simulink model "Unipolar_Bipolar_Sine_PWM_inverter"  (R2024b)
settings: Solver=VariableStepAuto  StartTime=0.0  StopTime=100e-3  RelTol=1e-3
libraries: spsMosfetLib x8, spsDCVoltageSourceLib x2, spsSeriesRLCBranchLib x2, spsTriangleGeneratorLib x2, spsVoltageMeasurementLib x2, sps_lib x1
settings Model: Creator=PRASHANTH  LastModifiedBy=PRASHANTH
settings DataIOCC: SaveOutput=off  SignalLogging=off  DSMLogging=off  ReturnWorkspaceOutputs=off  LoggingToFile=on

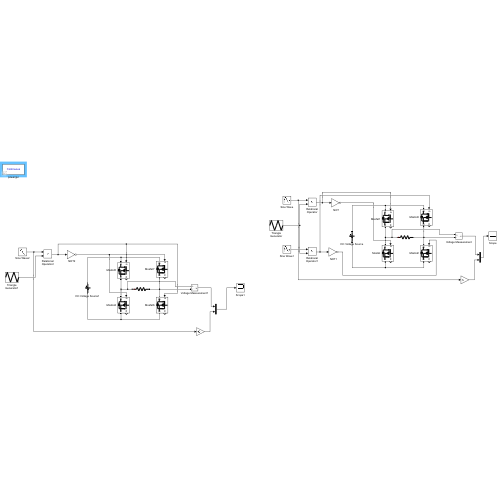
[thumbnail: Simulink's stored preview of the top-level diagram]
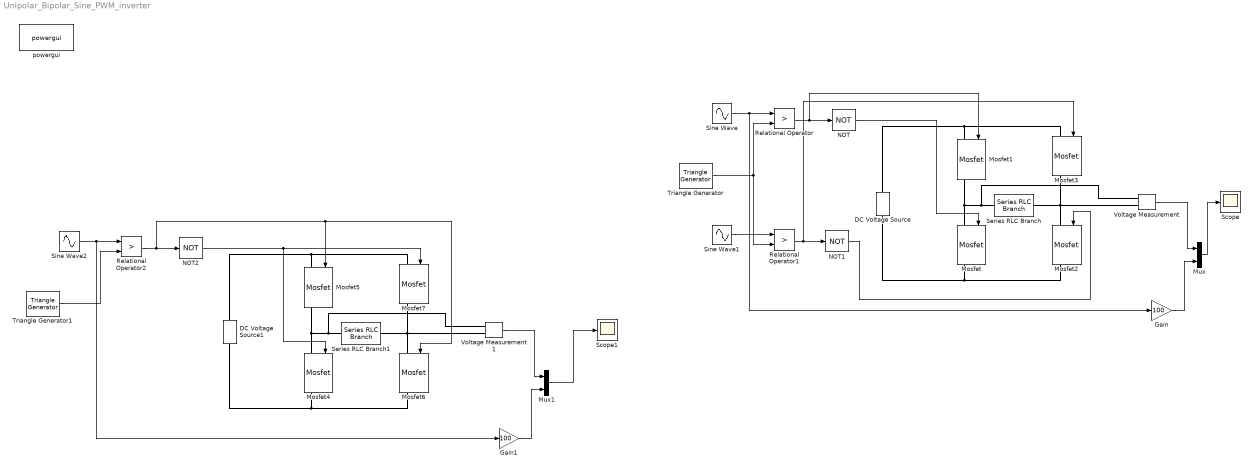
== system Unipolar_Bipolar_Sine_PWM_inverter ==
  DC Voltage Source : spsDCVoltageSourceLib/DC Voltage Source  Amplitude=100  Measurements=None
  DC Voltage Source1 : spsDCVoltageSourceLib/DC Voltage Source  Amplitude=100  Measurements=None
  Gain : Gain  Gain=100
  Gain1 : Gain  Gain=100
  Mosfet{,1..7} (8 alike) : spsMosfetLib/Mosfet  Ron=0.1  Lon=0  Rd=0.01  Vfd=0  IC=0  Rs=1e5  Cs=inf  Measurements=on
  Mux : Mux  Inputs=2
  Mux1 : Mux  Inputs=2
  NOT : Logic  Operator=NOT  IconShape=distinctive  AllPortsSameDT=off  OutDataTypeStr=boolean
  NOT1 : Logic  Operator=NOT  IconShape=distinctive  AllPortsSameDT=off  OutDataTypeStr=boolean
  NOT2 : Logic  Operator=NOT  IconShape=distinctive  AllPortsSameDT=off  OutDataTypeStr=boolean
  Relational Operator : RelationalOperator  Operator=>  OutDataTypeStr=boolean  RndMeth=Simplest  InputSameDT=off
  Relational Operator1 : RelationalOperator  Operator=>  OutDataTypeStr=boolean  RndMeth=Simplest  InputSameDT=off
  Relational Operator2 : RelationalOperator  Operator=>  OutDataTypeStr=boolean  RndMeth=Simplest  InputSameDT=off
  Scope : Scope
  Scope1 : Scope
  Series RLC Branch : spsSeriesRLCBranchLib/Series RLC Branch  LConnTagsString=__new0  RConnTagsString=__new0  BranchType=R  Resistance=10  Inductance=1e-3  SetiL0=off  InitialCurrent=0  Capacitance=1e-6  Setx0=off  InitialVoltage=0  Measurements=None
  Series RLC Branch1 : spsSeriesRLCBranchLib/Series RLC Branch  LConnTagsString=__new0  RConnTagsString=__new0  BranchType=R  Resistance=10  Inductance=1e-3  SetiL0=off  InitialCurrent=0  Capacitance=1e-6  Setx0=off  InitialVoltage=0  Measurements=None
  Sine Wave : Sin  Frequency=2*pi*50  SampleTime=0
  Sine Wave1 : Sin  Frequency=pi  SampleTime=0
  Sine Wave2 : Sin  Frequency=2*pi*50  SampleTime=0
  Triangle Generator : spsTriangleGeneratorLib/Triangle Generator  Freq=1e3  Phase=90  Ts=0
  Triangle Generator1 : spsTriangleGeneratorLib/Triangle Generator  Freq=1e3  Phase=90  Ts=0
  Voltage Measurement : spsVoltageMeasurementLib/Voltage Measurement  PhasorSimulation=off  OutputType=Complex  PSBequivalent=0
  Voltage Measurement1 : spsVoltageMeasurementLib/Voltage Measurement  PhasorSimulation=off  OutputType=Complex  PSBequivalent=0
  powergui : sps_lib/powergui  Priority=1  SimulationMode=Continuous  SampleTime=50e-6  frequency=60  Iterations=50  frequencyindice=0  Pbase=100e6  ErrMax=1e-4  UnitsV=kV  UnitsW=MW  buscounter=0  FunctionMessages=off  echomessages=off  EnableUseOfTLC=off  CurrentSourceSwitches=off  DisableSnubberDevices=off  DisableRonSwitches=off  DisableVfSwitches=off  DisplayEquations=off  AutomaticDiscreteSolvers=off  SolverType=Tustin/Backward Euler (TBE)  Interpol=off  ExternalGateDelay=off  methode=off  Ts=100  x0status=blocks  SPID=on  SwTol=0  HookPort=off  NonlinearTolerance=1e-4  nMaxIteration=100  ContinueOnMaxIteration=off  RestoreLinks=warning  ResistiveCurrentMeasurement=off  Frange=[0:2:500]  Ylog=off  Xlog=on  ShowGrid=off  save=off  variable=ZData  structure=0  ZoomFFT=off  StartTime=0.0  cycles=1  DisplayStyle=1  fundamental=60  FreqAxis=off  MaxFrequency=1000  frequencyindicesteady=1  RmsSteady=1  display=off
  wires:
  Sine Wave/1 -> Gain/1, Relational Operator/1
  Sine Wave1/1 -> Relational Operator1/1
  Triangle Generator/1 -> Relational Operator/2, Relational Operator1/2
  Relational Operator/1 -> Mosfet1/1, NOT/1
  NOT/1 -> Mosfet/1
  Relational Operator1/1 -> Mosfet3/1, NOT1/1
  NOT1/1 -> Mosfet2/1
  Gain/1 -> Mux/2
  Voltage Measurement/1 -> Mux/1
  Mux/1 -> Scope/1
  Triangle Generator1/1 -> Relational Operator2/2
  Mux1/1 -> Scope1/1
  Sine Wave2/1 -> Gain1/1, Relational Operator2/1
  Relational Operator2/1 -> Mosfet6/1, Mosfet5/1, NOT2/1
  NOT2/1 -> Mosfet7/1, Mosfet4/1
  Voltage Measurement1/1 -> Mux1/1
  Gain1/1 -> Mux1/2
  connections:
  DC Voltage Source/RConn1 -- Mosfet1/LConn1 -- Mosfet3/LConn1
  Mosfet1/RConn1 -- Voltage Measurement/LConn1 -- Series RLC Branch/LConn1 -- Mosfet/LConn1
  Mosfet3/RConn1 -- Series RLC Branch/RConn1 -- Voltage Measurement/LConn2 -- Mosfet2/LConn1
  Mosfet2/RConn1 -- Mosfet/RConn1 -- DC Voltage Source/LConn1
  DC Voltage Source1/LConn1 -- Mosfet4/RConn1 -- Mosfet6/RConn1
  Mosfet7/LConn1 -- Mosfet5/LConn1 -- DC Voltage Source1/RConn1
  Mosfet4/LConn1 -- Mosfet5/RConn1 -- Voltage Measurement1/LConn1 -- Series RLC Branch1/LConn1
  Mosfet6/LConn1 -- Series RLC Branch1/RConn1 -- Voltage Measurement1/LConn2 -- Mosfet7/RConn1
